simulink model "DC_Motor_Model"  (R2024b)
settings: Solver=VariableStepAuto  StartTime=0.0  StopTime=0.4  RelTol=1e-3
values from neighbouring files (symbols this model uses):
  B = 0    [DC_Motor_Project.m]
  J = 0.00252    [DC_Motor_Project.m]
  Kt = Te_rated / Ia_rated    (= 0.424752712124)    [DC_Motor_Project.m]
  La = 1.7e-3    (= 0.0017)    [DC_Motor_Project.m]
  Ra = 0.26    [DC_Motor_Project.m]
settings Model: Creator=LEGION  LastModifiedBy=LEGION

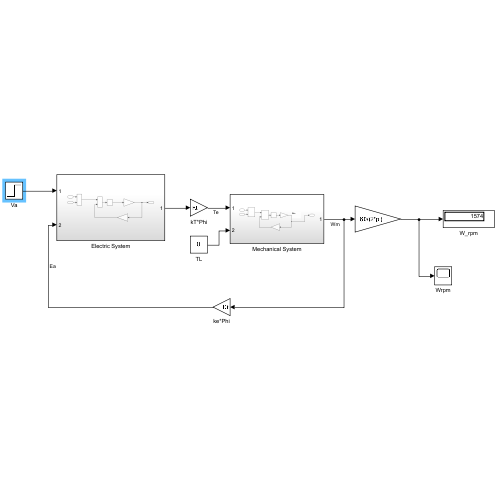
[thumbnail: Simulink's stored preview of the top-level diagram]
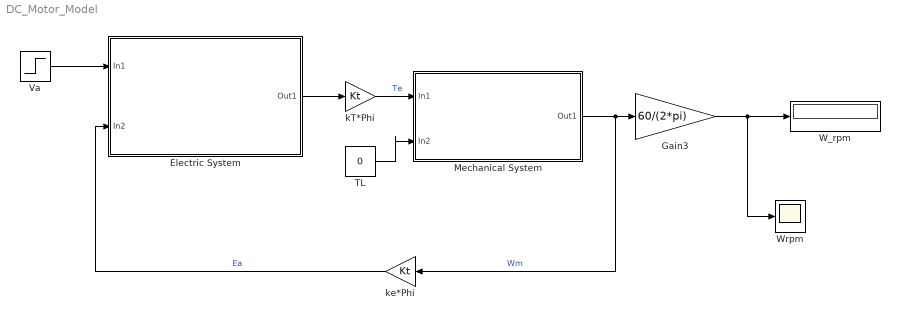
== system DC_Motor_Model ==
  Electric System : Subsystem
  Gain3 : Gain  Gain=60/(2*pi)
  Mechanical System : Subsystem
  TL : Constant  Value=0
  Va : Step  Time=0.05  After=70  SampleTime=0
  W_rpm : Display
  Wrpm : Scope
  kT*Phi : Gain  Gain=Kt
  ke*Phi : Gain  Gain=Kt
  wires:
  Electric System/1(Out1) -> kT*Phi/1
  Va/1 -> Electric System/1(In1)
  Gain3/1 -> Wrpm/1, W_rpm/1
  Mechanical System/1(Out1) -> ke*Phi/1, Gain3/1  "Wm"
  kT*Phi/1 -> Mechanical System/1(In1)  "Te"
  TL/1 -> Mechanical System/2(In2)
  ke*Phi/1 -> Electric System/2(In2)  "Ea"

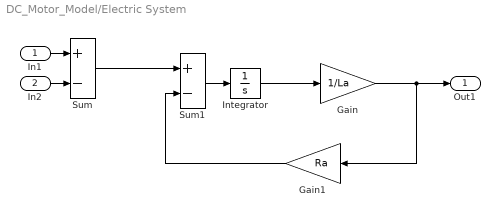
== system DC_Motor_Model/Electric System ==
  In1 : Inport
  In2 : Inport  Port=2
  Gain : Gain  Gain=1/La
  Gain1 : Gain  Gain=Ra
  Integrator : Integrator
  Sum : Sum  Inputs=+-
  Sum1 : Sum  Inputs=+-
  Out1 : Outport
  wires:
  Sum1/1 -> Integrator/1
  In1/1 -> Sum/1
  Gain1/1 -> Sum1/2
  Gain/1 -> Out1/1, Gain1/1
  Sum/1 -> Sum1/1
  Integrator/1 -> Gain/1
  In2/1 -> Sum/2

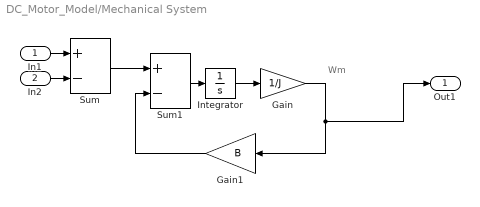
== system DC_Motor_Model/Mechanical System ==
  note: Wm
  In1 : Inport
  In2 : Inport  Port=2
  Gain : Gain  Gain=1/J
  Gain1 : Gain  Gain=B
  Integrator : Integrator
  Sum : Sum  Inputs=+-
  Sum1 : Sum  Inputs=+-
  Out1 : Outport
  wires:
  Gain/1 -> Out1/1, Gain1/1
  Sum1/1 -> Integrator/1
  Sum/1 -> Sum1/1
  In1/1 -> Sum/1
  Gain1/1 -> Sum1/2
  Integrator/1 -> Gain/1
  In2/1 -> Sum/2
